simulink model "r4_pfb_fir"  (Simulink 7.0)
settings: Solver=FixedStepDiscrete  SolverMode=SingleTasking  StartTime=0.0  StopTime=10.0  RelTol=1e-3
undefined symbols (not defined in the file): pfb_coefs
libraries: xbsIndex_r4 x385, xps_library x1
(part 2 of 27)

== system r4_pfb_fir/fir_1 ==
  in : Inport  OutDataType=sfix(16)  OutScaling=2^0
  sync_in : Inport  Port=2  OutDataType=sfix(16)  OutScaling=2^0
  Constant : xbsIndex_r4/Constant  arith_type=Unsigned  const=0  n_bits=34  bin_pt=0  explicit_period=on  period=1  equ=P=C  opselect=C  inp2=PCIN>>17  opr=+  inp1=P  carry=CIN  dbl_ovrd=off  block_type=constant
  fir_quantize : Subsystem  mask(FIR Filter Quantizer){n_bits_s=17, bin_pt_s=15, n_bits_o=9, bin_pt_o=7}
      mask prompts: n_bits_s "Number of Bits In"; bin_pt_s "Binary Point In"; n_bits_o "Number of Bits Out"; bin_pt_o "Binary Point Out"
      mask help: A Finite Impluse Response Filter ouput quantizer. This FIR filter output quantizer rounds the sum_in value to the precision specified by n_bits and bin_pt. Overflow wraps, but quantization rounds to even if input binary point is greater than output binary point, otherwise quantization tuncates.
      settings: AttributesFormatString=|
      | 17_15 in
      | 9_7 out
      | round even
      mask Help:
      | <pre>
      | Description::
      | 
      | A Finite Impluse Response Filter ouput quantizer.  This FIR filter output quantizer
      | rounds the sum_in value to the precision specified by n_bits and bin_pt.
      | 
      | Overflow wraps, but quantization rounds to even if input binary point is greater
      | than output binary point, otherwise quantization tuncates.
      | 
      | Mask Parameters::
      | 
      | Number of Bits In (n_bits_s): Specifies the width of the sum_in input.
      | 
      | Binary Point In (bin_pt_s): Specifies the binary point of the sum_in input.
      | 
      | Number of Bits Out (n_bits_o): Specifies the width of the output (overflow wraps).
      | 
      | Binary Point Out (bin_pt_o): Specifies the binary point of the output (quantization rounds to even
      | if input binary point is greater than output binary point, othersie quantization truncates).
      | </pre>
  fir_tap_1 : Subsystem  mask(FIR Filter Tap (Real Coefficients)){delay=1024, coef=[7.55822333239443e-005;0.000226337373781674;0.000376546527419557;0.000526209439676531;0.000675325864794748;0.000823895565799559;0.000971918314479012;0.00111939389136366;0.00126632208570627;0.00141270269546109;0.00155853552726339;0.00170382039640892;0.00184855712683285;0.00199274555108931;0.00213638551033019;0.0022794768542842;0.00242201944123601;0.00256401313800475;0.00270545781992298;0.00284635337081542;0.00298669968297734;0.00312649665715319;0.00326574420251518;0.00340444223664131;0.00354259068549404;0.00368018948339813;0.00381723857301899;0.00395373790534074;0.00408968743964404;0.00422508714348402;0.00435993699266828;0.00449423697123439;0.00462798707142765;0.00476118729367882;0.00489383764658139;0.00502593814686929;0.00515748881939405;0.00528848969710218;0.00541894082101253;0.00554884224019323;0.00567819401173886;0.00580699620074764;0.00593524888029807;0.006062952131426;0.0061901060431015;0.00631671071220536;0.00644276624350604;0.00656827274963604;0.00669323035106852;0.00681763917609391;0.00694149936079604;0.00706481104902866;0.00718757439239176;0.00730978955020755;0.00743145668949677;0.00755257598495482;0.00767314761892755;0.00779317178138749;0.00791264866990946;0.00803157848964654;0.00814996145330591;0.00826779778112436;0.00838508770084402;0.00850183144768805;0.00861802926433593;0.00873368140089908;0.00884878811489629;0.00896334967122888;0.00907736634215623;0.00919083840727075;0.00930376615347321;0.0094161498749479;0.00952798987313748;0.00963928645671813;0.00975003994157455;0.00986025065077467;0.00996991891454458;0.0100790450702434;0.0101876294623378;0.0102956724423769;0.0104031743689668;0.010510135607745;0.0106165565313551;0.0107224375194214;0.0108277789585228;0.010932581242168;0.0110368447707688;0.0111405699516152;0.0112437571988492;0.0113464069334393;0.0114485195831541;0.0115500955825369;0.0116511353728793;0.0117516394021958;0.0118516081251968;0.0119510420032635;0.012049941504421;0.0121483071033125;0.0122461392811728;0.0123434385258024;0.0124402053315406;0.0125364401992397;0.0126321436362382;0.0127273161563346;0.0128219582797607;0.0129160705331552;0.0130096534495371;0.013102707568279;0.0131952334350806;0.0132872316019417;0.013378702627136;0.0134696470751837;0.0135600655168253;0.0136499585289943;0.0137393266947904;0.0138281706034528;0.0139164908503332;0.0140042880368685;0.0140915627705541;0.0141783156649169;0.0142645473394878;0.0143502584197752;0.014435449537237;0.0145201213292544;0.0146042744391039;0.0146879095159304;0.0147710272147199;0.014853628196272;0.014935713127173;0.0150172826797681;0.0150983375321339;0.0151788783680517;0.0152589058769791;0.0153384207540233;0.0154174236999132;0.0154959154209719;0.0155738966290892;0.015651368041694;0.0157283303817268;0.0158047843776117;0.0158807307632293;0.0159561702778886;0.0160311036662993;0.0161055316785444;0.016179455070052;0.0162528746015679;0.0163257910391276;0.0163982051540287;0.0164701177228029;0.0165415295271879;0.0166124413541001;0.0166828539956064;0.016752768248896;0.0168221849162531;0.0168911048050285;0.0169595287276116;0.0170274575014029;0.0170948919487855;0.0171618328970972;0.0172282811786028;0.0172942376304655;0.0173597030947194;0.0174246784182411;0.0174891644527217;0.0175531620546388;0.0176166720852282;0.0176796954104559;0.01774223290099;0.0178042854321725;0.0178658538839913;0.0179269391410516;0.0179875420925484;0.0180476636322377;0.0181073046584087;0.0181664660738554;0.0182251487858485;0.0182833537061072;0.018341081750771;0.0183983338403711;0.018455110899803;0.0185114138582973;0.0185672436493922;0.0186226012109047;0.0186774874849029;0.0187319034176773;0.0187858499597128;0.0188393280656603;0.0188923386943085;0.0189448828085557;0.0189969613753813;0.0190485753658179;0.0190997257549227;0.0191504135217495;0.0192006396493202;0.0192504051245967;0.0192997109384527;0.019348558085645;0.0193969475647859;0.0194448803783146;0.0194923575324687;0.0195393800372564;0.0195859489064282;0.0196320651574482;0.0196777298114666;0.0197229438932907;0.0197677084313573;0.0198120244577041 ...(+15786 chars)], n_bits_c=9, bin_pt_c=8, n_bits_d=8, bin_pt_d=7, n_bits_s=17, bin_pt_s=15, coef_bram=on, delay_bram=on, mult_latency=3, add_latency=1, add_bypass=on}
      mask prompts: delay "Tap Delay"; coef "Tap Coefficient(s)"; n_bits_c "Number of Coefficient Bits"; bin_pt_c "Coefficient Binary Point"; n_bits_d "Number of Data Bits"; bin_pt_d "Data Binary Point"; n_bits_s "Number of Sum Bits"; bin_pt_s "Sum Binary Point"; coef_bram "Use BRAM for Coefficients"; delay_bram "Use BRAM for Delay"; mult_latency "Multiplier Latency"; add_latency "Adder Latency"; add_bypass "Bypass Adder"
      mask help: A Finite Impluse Response Filter tap with real coefficients. This FIR filter tap does not have provisions for folding the input sequence to improve multiplier efficiency, so it is suboptimal for "regular" (i.e. non-WOLA) FIR filters. It is intended primarily for WOLA (Weighted OverLap Add) FIR filters.
      settings: AttributesFormatString=|
      | delay 1024 in bram
      | 1024 coefs in bram\nno adder
      mask Help:
      | <pre>
      | Description::
      | 
      | A Finite Impluse Response Filter tap with real coefficients.
      | 
      | This Finite Impluse Response Filter tap is designed to be daisy chained together
      | to form a multi-tap FIR filter.  This FIR filter tap does not have provisions for folding the input
      | sequence to improve multiplier efficiency, so it is suboptimal for "regular" (i.e. non-WOLA)
      | FIR filters.  It is intended primarily for WOLA (Weighted OverLap Add) FIR filters.
      | 
      | Mask Parameters::
      | 
      | Tap Delay (delay):  The inter-tap delay (the N in "z^-N").  For a regular FIR filter, this will be 1.
      | 
      | Tap Coefficiant(s) (coef): The coefficient(s) for this tap.  For a regular FIR filter, this will be a
      | single number.  For a WOLA (Weighted OverLap Add) filter, this will be a vector of numbers.
      | Usually, delay==length(coef), but this is not required.  These should be specified as doubles.
      | They will be rounded and saturated according to the specified number of bits (n_bits_c) and
      | binary point (bin_pt_c).
      | 
      | Number of Coefficient Bits (n_bits_c): The number of bits used for the fixed point binary
      | representation of the coefficient(s).
      | 
      | Coefficient Binary Point (bin_pt_c): The binary point of the fixed point binary representation
      | of the coefficient(s).
      | 
      | Number of Data Bits (n_bits_d): The number of bits for real/imaginary components of the data.
      | 
      | Data Binary Point (bin_pt_d): The binary point for real/imaginary components of the data.
      | 
      | Number of Sum Bits (n_bits_s): Specifies the width of the sum (overflow wraps).
      | 
      | Sum Binary Point (bin_pt_s): Specifies the binary point of the sum (quantization truncates).
      | 
      | Use BRAM for Delay (delay_bram): Check this checkbox to implement the delay using BRAM.
      | If unchecked, the delay will be implemented using SLR16 elements (i.e. slices).
      | 
      | Use BRAM for Coefficients (coef_bram): Check this checkbox to store the coefficients in BRAM.
      | If unchecked, the coefficients will be stored in distributed memory (i.e. slices).
      | This is only relevant is length(coef) is greater than 1; otherwise, a constant block is used.
      | 
      | Multiplier Latency (mult_latency): Latency to use for the underlying multiplier.
      | 
      | Adder Latency (add_latency): Latency to use for the underlying adder.
      | 
      | Adder Bypass (add_bypass): Check this checkbox to bypass the adder.
      | Typically used for the first tap of a multi-tap FIR filter.
      | </pre>
  fir_tap_2 : Subsystem  mask(FIR Filter Tap (Real Coefficients)){delay=1024, coef=[-0.000375660323525046;-0.00112528207646786;-0.00187263770065757;-0.00261772609063303;-0.00336054616203061;-0.00410109685156988;-0.00483937711704019;-0.00557538593728603;-0.00630912231219222;-0.00704058526266978;-0.00776977383064064;-0.00849668707902262;-0.00922132409171369;-0.00994368397357705;-0.0106637658504249;-0.0113815688690025;-0.0120970921969721;-0.0128103350228962;-0.0135212965562215;-0.0142299760272615;-0.0149363726871797;-0.0156404858079725;-0.0163423146824514;-0.0170418586242254;-0.0177391169676835;-0.0184340890679761;-0.0191267743009973;-0.0198171720633655;-0.0205052817724058;-0.0211911028661302;-0.0218746348032188;-0.0225558770630009;-0.0232348291454347;-0.0239114905710882;-0.0245858608811188;-0.0252579396372536;-0.0259277264217688;-0.0265952208374693;-0.0272604225076676;-0.0279233310761635;-0.0285839462072226;-0.0292422675855545;-0.0298982949162921;-0.0305520279249694;-0.0312034663574997;-0.031852609980153;-0.0324994585795345;-0.0331440119625613;-0.0337862699564402;-0.0344262324086442;-0.0350638991868898;-0.0356992701791137;-0.0363323452934489;-0.0369631244582015;-0.0375916076218262;-0.0382177947529027;-0.0388416858401109;-0.0394632808922069;-0.0400825799379981;-0.0406995830263182;-0.0413142902260021;-0.0419267016258609;-0.0425368173346564;-0.0431446374810749;-0.0437501622137022;-0.0443533917009969;-0.0449543261312647;-0.0455529657126312;-0.0461493106730163;-0.0467433612601067;-0.047335117741329;-0.0479245804038229;-0.0485117495544134;-0.0490966255195838;-0.0496792086454471;-0.0502594992977191;-0.0508374978616896;-0.0514132047421944;-0.0519866203635867;-0.0525577451697087;-0.0531265796238626;-0.0536931242087811;-0.0542573794265993;-0.0548193457988244;-0.0553790238663066;-0.0559364141892089;-0.0564915173469777;-0.0570443339383125;-0.0575948645811356;-0.0581431099125613;-0.058689070588866;-0.0592327472854569;-0.0597741406968409;-0.0603132515365938;-0.0608500805373288;-0.0613846284506648;-0.0619168960471949;-0.0624468841164546;-0.0629745934668896;-0.0635000249258237;-0.064023179339426;-0.0645440575726791;-0.0650626605093458;-0.0655789890519362;-0.0660930441216749;-0.0666048266584676;-0.0671143376208679;-0.067621577986043;-0.0681265487497408;-0.0686292509262558;-0.0691296855483946;-0.0696278536674418;-0.0701237563531258;-0.0706173946935843;-0.071108769795329;-0.071597882783211;-0.0720847348003859;-0.0725693270082785;-0.0730516605865468;-0.0735317367330474;-0.0740095566637989;-0.0744851216129466;-0.0749584328327259;-0.0754294915934268;-0.0758982991833568;-0.0763648569088048;-0.0768291660940042;-0.0772912280810962;-0.0777510442300928;-0.0782086159188393;-0.0786639445429775;-0.0791170315159078;-0.0795678782687517;-0.0800164862503141;-0.0804628569270452;-0.0809069917830028;-0.0813488923198131;-0.0817885600566336;-0.0822259965301136;-0.0826612032943558;-0.0830941819208773;-0.0835249339985711;-0.0839534611336661;-0.0843797649496887;-0.0848038470874227;-0.0852257092048699;-0.0856453529772106;-0.0860627800967632;-0.0864779922729447;-0.0868909912322302;-0.0873017787181127;-0.0877103564910625;-0.0881167263284868;-0.0885208900246886;-0.0889228493908263;-0.0893226062548723;-0.0897201624615717;-0.0901155198724016;-0.0905086803655288;-0.0908996458357691;-0.0912884181945446;-0.0916749993698427;-0.0920593913061736;-0.0924415959645284;-0.0928216153223364;-0.0931994513734234;-0.0935751061279683;-0.0939485816124612;-0.09431987986966;-0.0946890029585477;-0.0950559529542894;-0.0954207319481889;-0.0957833420476455;-0.0961437853761105;-0.0965020640730433;-0.0968581802938682;-0.0972121362099301;-0.0975639340084509;-0.0979135758924848;-0.0982610640808748;-0.0986064008082076;-0.0989495883247697;-0.0992906288965024;-0.0996295248049575;-0.0999662783472516;-0.100300891836022;-0.100633367599381;-0.100963707980872;-0.101291915339421;-0.101617992049296;-0.101941940500055;-0.102263763096507;-0.102583462258662;-0.102901040421687;-0.103216500035856;-0.103529843566511;-0.103841073494009;-0.104150192313679;-0.104457202535775;-0.104762106685429 ...(+16057 chars)], n_bits_c=9, bin_pt_c=8, n_bits_d=8, bin_pt_d=7, n_bits_s=17, bin_pt_s=15, coef_bram=on, delay_bram=on, mult_latency=3, add_latency=1, add_bypass=off}
      mask prompts: delay "Tap Delay"; coef "Tap Coefficient(s)"; n_bits_c "Number of Coefficient Bits"; bin_pt_c "Coefficient Binary Point"; n_bits_d "Number of Data Bits"; bin_pt_d "Data Binary Point"; n_bits_s "Number of Sum Bits"; bin_pt_s "Sum Binary Point"; coef_bram "Use BRAM for Coefficients"; delay_bram "Use BRAM for Delay"; mult_latency "Multiplier Latency"; add_latency "Adder Latency"; add_bypass "Bypass Adder"
      mask help: A Finite Impluse Response Filter tap with real coefficients. This FIR filter tap does not have provisions for folding the input sequence to improve multiplier efficiency, so it is suboptimal for "regular" (i.e. non-WOLA) FIR filters. It is intended primarily for WOLA (Weighted OverLap Add) FIR filters.
      settings: AttributesFormatString=|
      | delay 1024 in bram
      | 1024 coefs in bram
      mask Help:
      | <pre>
      | Description::
      | 
      | A Finite Impluse Response Filter tap with real coefficients.
      | 
      | This Finite Impluse Response Filter tap is designed to be daisy chained together
      | to form a multi-tap FIR filter.  This FIR filter tap does not have provisions for folding the input
      | sequence to improve multiplier efficiency, so it is suboptimal for "regular" (i.e. non-WOLA)
      | FIR filters.  It is intended primarily for WOLA (Weighted OverLap Add) FIR filters.
      | 
      | Mask Parameters::
      | 
      | Tap Delay (delay):  The inter-tap delay (the N in "z^-N").  For a regular FIR filter, this will be 1.
      | 
      | Tap Coefficiant(s) (coef): The coefficient(s) for this tap.  For a regular FIR filter, this will be a
      | single number.  For a WOLA (Weighted OverLap Add) filter, this will be a vector of numbers.
      | Usually, delay==length(coef), but this is not required.  These should be specified as doubles.
      | They will be rounded and saturated according to the specified number of bits (n_bits_c) and
      | binary point (bin_pt_c).
      | 
      | Number of Coefficient Bits (n_bits_c): The number of bits used for the fixed point binary
      | representation of the coefficient(s).
      | 
      | Coefficient Binary Point (bin_pt_c): The binary point of the fixed point binary representation
      | of the coefficient(s).
      | 
      | Number of Data Bits (n_bits_d): The number of bits for real/imaginary components of the data.
      | 
      | Data Binary Point (bin_pt_d): The binary point for real/imaginary components of the data.
      | 
      | Number of Sum Bits (n_bits_s): Specifies the width of the sum (overflow wraps).
      | 
      | Sum Binary Point (bin_pt_s): Specifies the binary point of the sum (quantization truncates).
      | 
      | Use BRAM for Delay (delay_bram): Check this checkbox to implement the delay using BRAM.
      | If unchecked, the delay will be implemented using SLR16 elements (i.e. slices).
      | 
      | Use BRAM for Coefficients (coef_bram): Check this checkbox to store the coefficients in BRAM.
      | If unchecked, the coefficients will be stored in distributed memory (i.e. slices).
      | This is only relevant is length(coef) is greater than 1; otherwise, a constant block is used.
      | 
      | Multiplier Latency (mult_latency): Latency to use for the underlying multiplier.
      | 
      | Adder Latency (add_latency): Latency to use for the underlying adder.
      | 
      | Adder Bypass (add_bypass): Check this checkbox to bypass the adder.
      | Typically used for the first tap of a multi-tap FIR filter.
      | </pre>
  fir_tap_3 : Subsystem  mask(FIR Filter Tap (Real Coefficients)){delay=1024, coef=[0.999999547662946;0.999995928971626;0.999988691616268;0.999977835651433;0.999963361158965;0.999945268247983;0.999923557054889;0.99989822774336;0.999869280504348;0.999836715556079;0.999800533144051;0.99976073354103;0.999717317047049;0.999670283989403;0.999619634722648;0.999565369628596;0.999507489116311;0.999445993622108;0.999380883609544;0.999312159569415;0.999239822019754;0.999163871505822;0.999084308600105;0.999001133902306;0.998914348039344;0.998823951665339;0.998729945461616;0.99863233013669;0.998531106426262;0.998426275093213;0.998317836927595;0.998205792746621;0.998090143394661;0.997970889743233;0.99784803269099;0.997721573163716;0.997591512114315;0.997457850522799;0.997320589396285;0.997179729768976;0.997035272702159;0.99688721928419;0.996735570630482;0.996580327883498;0.996421492212737;0.996259064814724;0.996093046912996;0.99592343975809;0.995750244627533;0.995573462825828;0.99539309568444;0.995209144561783;0.995021610843209;0.994830495940991;0.99463580129431;0.994437528369243;0.994235678658745;0.994030253682635;0.993821254987582;0.993608684147091;0.993392542761483;0.993172832457882;0.992949554890201;0.99272271173912;0.992492304712073;0.992258335543232;0.992020805993488;0.991779717850431;0.991535072928337;0.991286873068149;0.991035120137455;0.990779816030475;0.990520962668036;0.990258561997559;0.989992615993036;0.989723126655011;0.989450096010561;0.989173526113274;0.988893419043231;0.988609776906985;0.988322601837537;0.98803189599432;0.987737661563173;0.987439900756322;0.987138615812356;0.986833808996206;0.986525482599124;0.986213638938657;0.985898280358627;0.985579409229105;0.98525702794639;0.984931138932984;0.984601744637569;0.984268847534979;0.98393245012618;0.983592554938246;0.983249164524326;0.98290228146363;0.982551908361392;0.982198047848854;0.981840702583234;0.9814798752477;0.981115568551347;0.980747785229165;0.980376528042017;0.98000179977661;0.979623603245462;0.979241941286885;0.978856816764947;0.978468232569446;0.978076191615887;0.977680696845445;0.977281751224942;0.976879357746813;0.97647351942908;0.976064239315321;0.975651520474639;0.975235366001631;0.97481577901636;0.974392762664321;0.973966320116415;0.973536454568909;0.973103169243412;0.972666467386842;0.972226352271389;0.971782827194488;0.971335895478783;0.970885560472097;0.970431825547395;0.969974694102756;0.969514169561332;0.969050255371323;0.968582955005935;0.96811227196335;0.967638209766689;0.967160771963981;0.966679962128122;0.966195783856846;0.965708240772684;0.965217336522932;0.964723074779614;0.964225459239442;0.963724493623787;0.963220181678634;0.962712527174551;0.962201533906649;0.961687205694544;0.961169546382321;0.960648559838497;0.960124249955978;0.959596620652025;0.959065675868214;0.958531419570396;0.95799385574866;0.957452988417292;0.956908821614734;0.956361359403548;0.955810605870372;0.955256565125884;0.954699241304754;0.954138638565613;0.953574761091004;0.953007613087343;0.952437198784881;0.951863522437655;0.951286588323455;0.950706400743774;0.950122964023769;0.949536282512219;0.948946360581481;0.948353202627446;0.947756813069498;0.947157196350468;0.946554356936591;0.945948299317464;0.945339028005997;0.944726547538374;0.944110862474005;0.943491977395482;0.942869896908532;0.942244625641977;0.941616168247679;0.940984529400506;0.940349713798277;0.939711726161716;0.939070571234412;0.938426253782768;0.937778778595951;0.937128150485851;0.936474374287031;0.935817454856679;0.935157397074559;0.934494205842967;0.933827886086677;0.933158442752899;0.932485880811225;0.931810205253583;0.931131421094187;0.930449533369489;0.929764547138127;0.929076467480875;0.928385299500598;0.927691048322198;0.92699371909256;0.926293316980511;0.925589847176761;0.924883314893854;0.924173725366119;0.923461083849616;0.922745395622088;0.922026665982904;0.92130490025301;0.920580103774877;0.919852281912448;0.919121440051086;0.918387583597519;0.91765071797979;0.9169108486472;0.916167981070258;0.915422120740627;0.914673273171068;0.913921443895387;0.913166638468382 ...(+14460 chars)], n_bits_c=9, bin_pt_c=8, n_bits_d=8, bin_pt_d=7, n_bits_s=17, bin_pt_s=15, coef_bram=on, delay_bram=on, mult_latency=3, add_latency=1, add_bypass=off}
      mask prompts: delay "Tap Delay"; coef "Tap Coefficient(s)"; n_bits_c "Number of Coefficient Bits"; bin_pt_c "Coefficient Binary Point"; n_bits_d "Number of Data Bits"; bin_pt_d "Data Binary Point"; n_bits_s "Number of Sum Bits"; bin_pt_s "Sum Binary Point"; coef_bram "Use BRAM for Coefficients"; delay_bram "Use BRAM for Delay"; mult_latency "Multiplier Latency"; add_latency "Adder Latency"; add_bypass "Bypass Adder"
      mask help: A Finite Impluse Response Filter tap with real coefficients. This FIR filter tap does not have provisions for folding the input sequence to improve multiplier efficiency, so it is suboptimal for "regular" (i.e. non-WOLA) FIR filters. It is intended primarily for WOLA (Weighted OverLap Add) FIR filters.
      settings: AttributesFormatString=|
      | delay 1024 in bram
      | 1024 coefs in bram
      mask Help:
      | <pre>
      | Description::
      | 
      | A Finite Impluse Response Filter tap with real coefficients.
      | 
      | This Finite Impluse Response Filter tap is designed to be daisy chained together
      | to form a multi-tap FIR filter.  This FIR filter tap does not have provisions for folding the input
      | sequence to improve multiplier efficiency, so it is suboptimal for "regular" (i.e. non-WOLA)
      | FIR filters.  It is intended primarily for WOLA (Weighted OverLap Add) FIR filters.
      | 
      | Mask Parameters::
      | 
      | Tap Delay (delay):  The inter-tap delay (the N in "z^-N").  For a regular FIR filter, this will be 1.
      | 
      | Tap Coefficiant(s) (coef): The coefficient(s) for this tap.  For a regular FIR filter, this will be a
      | single number.  For a WOLA (Weighted OverLap Add) filter, this will be a vector of numbers.
      | Usually, delay==length(coef), but this is not required.  These should be specified as doubles.
      | They will be rounded and saturated according to the specified number of bits (n_bits_c) and
      | binary point (bin_pt_c).
      | 
      | Number of Coefficient Bits (n_bits_c): The number of bits used for the fixed point binary
      | representation of the coefficient(s).
      | 
      | Coefficient Binary Point (bin_pt_c): The binary point of the fixed point binary representation
      | of the coefficient(s).
      | 
      | Number of Data Bits (n_bits_d): The number of bits for real/imaginary components of the data.
      | 
      | Data Binary Point (bin_pt_d): The binary point for real/imaginary components of the data.
      | 
      | Number of Sum Bits (n_bits_s): Specifies the width of the sum (overflow wraps).
      | 
      | Sum Binary Point (bin_pt_s): Specifies the binary point of the sum (quantization truncates).
      | 
      | Use BRAM for Delay (delay_bram): Check this checkbox to implement the delay using BRAM.
      | If unchecked, the delay will be implemented using SLR16 elements (i.e. slices).
      | 
      | Use BRAM for Coefficients (coef_bram): Check this checkbox to store the coefficients in BRAM.
      | If unchecked, the coefficients will be stored in distributed memory (i.e. slices).
      | This is only relevant is length(coef) is greater than 1; otherwise, a constant block is used.
      | 
      | Multiplier Latency (mult_latency): Latency to use for the underlying multiplier.
      | 
      | Adder Latency (add_latency): Latency to use for the underlying adder.
      | 
      | Adder Bypass (add_bypass): Check this checkbox to bypass the adder.
      | Typically used for the first tap of a multi-tap FIR filter.
      | </pre>
  fir_tap_4 : Subsystem  mask(FIR Filter Tap (Real Coefficients)){delay=1024, coef=[0.000376226431598763;0.00113037704120664;0.00188679033646423;0.00264546512738635;0.00340640020282435;0.00416959433045314;0.00493504625675948;0.00570275470702945;0.00647271838533626;0.00724493597452914;0.00801940613622144;0.00879612751077952;0.00957509871731131;0.0103563183536561;0.0111397849963734;0.0119254972007329;0.0127134535007037;0.0135036524089452;0.0142960924167967;0.0150907719942678;0.0158876895900297;0.0166868436314057;0.0174882325243625;0.0182918546535009;0.0190977083820486;0.019905792051851;0.0207161039833637;0.0215286424756441;0.022343405806345;0.0231603922317064;0.0239795999865484;0.0248010272842649;0.0256246723168164;0.026450533254724;0.0272786082470629;0.0281088954214566;0.0289413928840709;0.0297760987196091;0.0306130109913055;0.0314521277409214;0.0322934469887399;0.0331369667335609;0.0339826849526973;0.0348305996019707;0.035680708615707;0.0365330099067331;0.0373875013663734;0.0382441808644464;0.0391030462492619;0.0399640953476175;0.0408273259647971;0.0416927358845677;0.0425603228691775;0.0434300846593541;0.0443020189743029;0.0451761235117054;0.0460523959477181;0.0469308339369715;0.0478114351125697;0.0486941970860893;0.0495791174475793;0.0504661937655611;0.0513554235870291;0.0522468044374499;0.0531403338207642;0.0540360092193872;0.0549338280942094;0.055833787884598;0.0567358860083988;0.0576401198619378;0.0585464868200229;0.0594549842359465;0.0603656094414881;0.0612783597469165;0.062193232440993;0.0631102247909746;0.0640293340426176;0.0649505574201807;0.0658738921264291;0.066799335342639;0.0677268842286013;0.0686565359226264;0.069588287541549;0.0705221361807334;0.0714580789140785;0.0723961127940227;0.0733362348515507;0.0742784420961991;0.0752227315160621;0.0761691000777984;0.0771175447266376;0.0780680623863875;0.0790206499594406;0.0799753043267821;0.0809320223479969;0.081890800861278;0.0828516366834338;0.0838145266098974;0.0847794674147343;0.0857464558506515;0.0867154886490061;0.0876865625198155;0.0886596741517658;0.0896348202122217;0.0906119973472373;0.091591202181565;0.0925724313186671;0.0935556813407251;0.094540948808652;0.0955282302621025;0.0965175222194845;0.0975088211779706;0.0985021236135104;0.0994974259808421;0.100494724713505;0.10149401622385;0.102495296903059;0.103498563121147;0.104503811226986;0.105511037548312;0.106520238391741;0.107531410042783;0.108544548765853;0.109559650804292;0.110576712380376;0.111595729695331;0.112616698929352;0.113639616241614;0.114664477770291;0.11569127963257;0.116720017924666;0.117750688721843;0.118783288078423;0.11981781202781;0.120854256582503;0.121892617734113;0.122932891453382;0.123975073690202;0.125019160373628;0.126065147411903;0.12711303069247;0.128162806081993;0.129214469426379;0.13026801655079;0.131323443259671;0.132380745336762;0.133439918545122;0.134500958627148;0.135563861304595;0.136628622278597;0.137695237229687;0.138763701817818;0.139834011682386;0.140906162442248;0.141980149695748;0.143055969020734;0.144133615974584;0.145213086094228;0.146294374896168;0.147377477876504;0.148462390510953;0.149549108254878;0.150637626543306;0.151727940790955;0.152820046392257;0.153913938721383;0.155009613132265;0.156107064958625;0.157206289513996;0.158307282091748;0.159410037965114;0.160514552387217;0.161620820591094;0.162728837789721;0.163838599176042;0.164950099922995;0.166063335183536;0.167178300090671;0.168294989757478;0.169413399277137;0.170533523722959;0.171655358148411;0.172778897587147;0.173904137053034;0.175031071540182;0.176159696022971;0.177290005456083;0.178421994774532;0.179555658893686;0.180690992709306;0.181827991097572;0.182966648915113;0.184106960999035;0.185248922166959;0.186392527217044;0.187537770928023;0.188684648059233;0.189833153350645;0.190983281522898;0.192135027277332;0.193288385296015;0.194443350241782;0.195599916758264;0.196758079469921;0.197917832982076;0.199079171880949;0.200242090733689;0.201406584088409;0.202572646474221;0.203740272401268;0.204909456360757;0.206080192825002;0.207252476247449;0.208426301062716;0.209601661686629 ...(+14467 chars)], n_bits_c=9, bin_pt_c=8, n_bits_d=8, bin_pt_d=7, n_bits_s=17, bin_pt_s=15, coef_bram=on, delay_bram=on, mult_latency=3, add_latency=1, add_bypass=off}
      mask prompts: delay "Tap Delay"; coef "Tap Coefficient(s)"; n_bits_c "Number of Coefficient Bits"; bin_pt_c "Coefficient Binary Point"; n_bits_d "Number of Data Bits"; bin_pt_d "Data Binary Point"; n_bits_s "Number of Sum Bits"; bin_pt_s "Sum Binary Point"; coef_bram "Use BRAM for Coefficients"; delay_bram "Use BRAM for Delay"; mult_latency "Multiplier Latency"; add_latency "Adder Latency"; add_bypass "Bypass Adder"
      mask help: A Finite Impluse Response Filter tap with real coefficients. This FIR filter tap does not have provisions for folding the input sequence to improve multiplier efficiency, so it is suboptimal for "regular" (i.e. non-WOLA) FIR filters. It is intended primarily for WOLA (Weighted OverLap Add) FIR filters.
      settings: AttributesFormatString=|
      | delay 1024 in bram
      | 1024 coefs in bram
      mask Help:
      | <pre>
      | Description::
      | 
      | A Finite Impluse Response Filter tap with real coefficients.
      | 
      | This Finite Impluse Response Filter tap is designed to be daisy chained together
      | to form a multi-tap FIR filter.  This FIR filter tap does not have provisions for folding the input
      | sequence to improve multiplier efficiency, so it is suboptimal for "regular" (i.e. non-WOLA)
      | FIR filters.  It is intended primarily for WOLA (Weighted OverLap Add) FIR filters.
      | 
      | Mask Parameters::
      | 
      | Tap Delay (delay):  The inter-tap delay (the N in "z^-N").  For a regular FIR filter, this will be 1.
      | 
      | Tap Coefficiant(s) (coef): The coefficient(s) for this tap.  For a regular FIR filter, this will be a
      | single number.  For a WOLA (Weighted OverLap Add) filter, this will be a vector of numbers.
      | Usually, delay==length(coef), but this is not required.  These should be specified as doubles.
      | They will be rounded and saturated according to the specified number of bits (n_bits_c) and
      | binary point (bin_pt_c).
      | 
      | Number of Coefficient Bits (n_bits_c): The number of bits used for the fixed point binary
      | representation of the coefficient(s).
      | 
      | Coefficient Binary Point (bin_pt_c): The binary point of the fixed point binary representation
      | of the coefficient(s).
      | 
      | Number of Data Bits (n_bits_d): The number of bits for real/imaginary components of the data.
      | 
      | Data Binary Point (bin_pt_d): The binary point for real/imaginary components of the data.
      | 
      | Number of Sum Bits (n_bits_s): Specifies the width of the sum (overflow wraps).
      | 
      | Sum Binary Point (bin_pt_s): Specifies the binary point of the sum (quantization truncates).
      | 
      | Use BRAM for Delay (delay_bram): Check this checkbox to implement the delay using BRAM.
      | If unchecked, the delay will be implemented using SLR16 elements (i.e. slices).
      | 
      | Use BRAM for Coefficients (coef_bram): Check this checkbox to store the coefficients in BRAM.
      | If unchecked, the coefficients will be stored in distributed memory (i.e. slices).
      | This is only relevant is length(coef) is greater than 1; otherwise, a constant block is used.
      | 
      | Multiplier Latency (mult_latency): Latency to use for the underlying multiplier.
      | 
      | Adder Latency (add_latency): Latency to use for the underlying adder.
      | 
      | Adder Bypass (add_bypass): Check this checkbox to bypass the adder.
      | Typically used for the first tap of a multi-tap FIR filter.
      | </pre>
  fir_tap_5 : Subsystem  mask(FIR Filter Tap (Real Coefficients)){delay=1024, coef=[-7.57186305694141e-005;-0.000227564945670749;-0.000379956430889435;-0.000532892796251757;-0.000686373742881339;-0.000840398962979647;-0.000994968139806186;-0.00115008094765919;-0.00130573705185642;-0.00146193610871559;-0.00161867776553536;-0.00177596166057639;-0.00193378742304204;-0.0020921546730598;-0.0022510630216622;-0.00241051207076825;-0.00257050141316491;-0.00273103063248833;-0.00289209930320557;-0.00305370699059638;-0.00321585325073467;-0.00337853763047057;-0.00354175966741245;-0.00370551888990871;-0.00386981481703025;-0.00403464695855241;-0.00420001481493748;-0.00436591787731722;-0.0045323556274752;-0.00469932753782952;-0.00486683307141569;-0.00503487168186923;-0.00520344281340873;-0.00537254590081901;-0.00554218036943399;-0.00571234563512023;-0.00588304110426002;-0.00605426617373492;-0.00622602023090949;-0.00639830265361464;-0.00657111281013151;-0.00674445005917552;-0.00691831374988003;-0.00709270322178053;-0.00726761780479901;-0.00744305681922785;-0.00761901957571464;-0.00779550537524631;-0.0079725135091339;-0.00815004325899737;-0.00832809389675017;-0.0085066646845843;-0.00868575487495546;-0.00886536371056795;-0.00904549042435999;-0.00922613423948933;-0.00940729436931827;-0.0095889700173997;-0.00977116037746245;-0.00995386463339719;-0.0101370819592425;-0.0103208115191707;-0.010505052467474;-0.0106898039485508;-0.0108750650968923;-0.0110608350370682;-0.0112471128837145;-0.011433897741519;-0.0116211887052088;-0.0118089848595372;-0.0119972852792704;-0.0121860890291751;-0.0123753951640054;-0.0125652027284904;-0.0127555107573218;-0.0129463182751411;-0.013137624296528;-0.0133294278259877;-0.0135217278579391;-0.013714523376703;-0.0139078133564902;-0.0141015967613896;-0.0142958725453573;-0.0144906396522044;-0.0146858970155864;-0.0148816435589916;-0.01507787819573;-0.0152745998289226;-0.0154718073514906;-0.0156694996461444;-0.0158676755853733;-0.016066334031435;-0.016265473836345;-0.0164650938418669;-0.016665192879502;-0.0168657697704791;-0.0170668233257453;-0.0172683523459559;-0.0174703556214645;-0.0176728319323143;-0.0178757800482282;-0.0180791987285998;-0.0182830867224842;-0.018487442768589;-0.0186922655952659;-0.0188975539205014;-0.0191033064519087;-0.019309521886719;-0.0195161989117731;-0.0197233362035136;-0.0199309324279764;-0.0201389862407831;-0.020347496287133;-0.0205564612017955;-0.0207658796091025;-0.0209757501229411;-0.0211860713467461;-0.0213968418734932;-0.0216080602856917;-0.0218197251553776;-0.022031835044107;-0.0222443885029495;-0.0224573840724814;-0.0226708202827797;-0.0228846956534157;-0.0230990086934489;-0.0233137579014212;-0.0235289417653507;-0.0237445587627263;-0.0239606073605024;-0.0241770860150929;-0.024393993172366;-0.0246113272676396;-0.0248290867256759;-0.025047269960676;-0.0252658753762764;-0.0254849013655432;-0.0257043463109681;-0.0259242085844644;-0.026144486547362;-0.0263651785504042;-0.026586282933743;-0.026807798026936;-0.0270297221489423;-0.0272520536081191;-0.0274747907022183;-0.0276979317183836;-0.0279214749331467;-0.0281454186124251;-0.0283697610115189;-0.0285945003751079;-0.0288196349372498;-0.029045162921377;-0.0292710825402948;-0.0294973919961793;-0.0297240894805752;-0.0299511731743939;-0.0301786412479123;-0.0304064918607708;-0.0306347231619722;-0.03086333328988;-0.0310923203722177;-0.0313216825260677;-0.0315514178578704;-0.0317815244634236;-0.0320120004278819;-0.0322428438257562;-0.0324740527209136;-0.0327056251665774;-0.0329375592053265;-0.0331698528690966;-0.0334025041791795;-0.0336355111462241;-0.0338688717702371;-0.0341025840405833;-0.0343366459359869;-0.0345710554245323;-0.0348058104636656;-0.0350409090001953;-0.0352763489702948;-0.035512128299503;-0.0357482449027266;-0.0359846966842419;-0.036221481537697;-0.036458597346114;-0.0366960419818909;-0.0369338133068049;-0.0371719091720144;-0.0374103274180622;-0.037649065874878;-0.0378881223617824;-0.038127494687489;-0.0383671806501086;-0.0386071780371525;-0.0388474846255361;-0.0390880981815831;-0.039329016461029;-0.0395702372090256 ...(+16053 chars)], n_bits_c=9, bin_pt_c=8, n_bits_d=8, bin_pt_d=7, n_bits_s=17, bin_pt_s=15, coef_bram=on, delay_bram=on, mult_latency=3, add_latency=1, add_bypass=off}
      mask prompts: delay "Tap Delay"; coef "Tap Coefficient(s)"; n_bits_c "Number of Coefficient Bits"; bin_pt_c "Coefficient Binary Point"; n_bits_d "Number of Data Bits"; bin_pt_d "Data Binary Point"; n_bits_s "Number of Sum Bits"; bin_pt_s "Sum Binary Point"; coef_bram "Use BRAM for Coefficients"; delay_bram "Use BRAM for Delay"; mult_latency "Multiplier Latency"; add_latency "Adder Latency"; add_bypass "Bypass Adder"
      mask help: A Finite Impluse Response Filter tap with real coefficients. This FIR filter tap does not have provisions for folding the input sequence to improve multiplier efficiency, so it is suboptimal for "regular" (i.e. non-WOLA) FIR filters. It is intended primarily for WOLA (Weighted OverLap Add) FIR filters.
      settings: AttributesFormatString=|
      | delay 1024 in bram
      | 1024 coefs in bram
      mask Help:
      | <pre>
      | Description::
      | 
      | A Finite Impluse Response Filter tap with real coefficients.
      | 
      | This Finite Impluse Response Filter tap is designed to be daisy chained together
      | to form a multi-tap FIR filter.  This FIR filter tap does not have provisions for folding the input
      | sequence to improve multiplier efficiency, so it is suboptimal for "regular" (i.e. non-WOLA)
      | FIR filters.  It is intended primarily for WOLA (Weighted OverLap Add) FIR filters.
      | 
      | Mask Parameters::
      | 
      | Tap Delay (delay):  The inter-tap delay (the N in "z^-N").  For a regular FIR filter, this will be 1.
      | 
      | Tap Coefficiant(s) (coef): The coefficient(s) for this tap.  For a regular FIR filter, this will be a
      | single number.  For a WOLA (Weighted OverLap Add) filter, this will be a vector of numbers.
      | Usually, delay==length(coef), but this is not required.  These should be specified as doubles.
      | They will be rounded and saturated according to the specified number of bits (n_bits_c) and
      | binary point (bin_pt_c).
      | 
      | Number of Coefficient Bits (n_bits_c): The number of bits used for the fixed point binary
      | representation of the coefficient(s).
      | 
      | Coefficient Binary Point (bin_pt_c): The binary point of the fixed point binary representation
      | of the coefficient(s).
      | 
      | Number of Data Bits (n_bits_d): The number of bits for real/imaginary components of the data.
      | 
      | Data Binary Point (bin_pt_d): The binary point for real/imaginary components of the data.
      | 
      | Number of Sum Bits (n_bits_s): Specifies the width of the sum (overflow wraps).
      | 
      | Sum Binary Point (bin_pt_s): Specifies the binary point of the sum (quantization truncates).
      | 
      | Use BRAM for Delay (delay_bram): Check this checkbox to implement the delay using BRAM.
      | If unchecked, the delay will be implemented using SLR16 elements (i.e. slices).
      | 
      | Use BRAM for Coefficients (coef_bram): Check this checkbox to store the coefficients in BRAM.
      | If unchecked, the coefficients will be stored in distributed memory (i.e. slices).
      | This is only relevant is length(coef) is greater than 1; otherwise, a constant block is used.
      | 
      | Multiplier Latency (mult_latency): Latency to use for the underlying multiplier.
      | 
      | Adder Latency (add_latency): Latency to use for the underlying adder.
      | 
      | Adder Bypass (add_bypass): Check this checkbox to bypass the adder.
      | Typically used for the first tap of a multi-tap FIR filter.
      | </pre>
  fir_tap_6 : Subsystem  mask(FIR Filter Tap (Real Coefficients)){delay=0, coef=[1.30229478472013e-005;3.90815624059165e-005;6.51573367774649e-005;9.12505128142159e-005;0.000117361332654004;0.000143490038707315;0.000169636873644433;0.000195802080382638;0.000221985902073233;0.000248188582088693;0.00027441036400972;0.000300651491612275;0.00032691220885466;0.000353192759864432;0.00037949338892544;0.000405814340464771;0.000432155859039685;0.000458518189324518;0.000484901576097635;0.000511306264228219;0.00053773249866318;0.000564180524413982;0.000590650586543436;0.000617142930152563;0.000643657800367275;0.000670195442325197;0.000696756101162392;0.00072334002200008;0.000749947449931329;0.000776578630007802;0.000803233807226332;0.000829913226515637;0.00085661713272294;0.000883345770600572;0.000910099384792634;0.000936878219821494;0.000963682520074419;0.000990512529790111;0.00101736849304526;0.00104425065374103;0.00107115925558966;0.00109809454210086;0.00112505675656834;0.00115204614205629;0.0011790629413858;0.00120610739712138;0.00123317975155729;0.00126028024670401;0.00128740912427467;0.0013145666256714;0.00134175299197172;0.00136896846391498;0.00139621328188859;0.00142348768591449;0.00145079191563545;0.00147812621030134;0.0015054908087556;0.00153288594942139;0.00156031187028796;0.00158776880889696;0.00161525700232871;0.00164277668718846;0.00167032809959269;0.00169791147515534;0.00172552704897407;0.00175317505561652;0.00178085572910654;0.00180856930291045;0.00183631600992321;0.00186409608245468;0.00189190975221584;0.001919757250305;0.00194763880719397;0.00197555465271432;0.00200350501604353;0.00203149012569121;0.00205951020948525;0.00208756549455806;0.00211565620733274;0.00214378257350922;0.00217194481805049;0.00220014316516874;0.00222837783831153;0.002256649060148;0.00228495705255503;0.00231330203660339;0.00234168423254391;0.00237010385979366;0.00239856113692212;0.00242705628163739;0.00245558951077227;0.0024841610402705;0.00251277108517291;0.00254141985960361;0.00257010757675613;0.00259883444887969;0.00262760068726523;0.00265640650223175;0.00268525210311237;0.00271413769824061;0.00274306349493657;0.00277202969949308;0.00280103651716193;0.00283008415214012;0.00285917280755598;0.00288830268545549;0.00291747398678844;0.00294668691139467;0.00297594165799033;0.00300523842415407;0.00303457740631335;0.00306395879973069;0.00309338279848989;0.00312284959548233;0.00315235938239325;0.00318191234968804;0.00321150868659852;0.00324114858110932;0.00327083221994408;0.00330055978855185;0.00333033147109343;0.00336014745042765;0.00339000790809786;0.00341991302431814;0.0034498629779598;0.00347985794653768;0.00350989810619665;0.00353998363169792;0.0035701146964056;0.00360029147227299;0.00363051412982916;0.00366078283816534;0.00369109776492143;0.00372145907627252;0.00375186693691537;0.00378232151005492;0.00381282295739088;0.00384337143910425;0.00387396711384388;0.00390461013871314;0.00393530066925641;0.00396603885944579;0.00399682486166768;0.00402765882670945;0.0040585409037462;0.00408947124032728;0.00412044998236316;0.00415147727411206;0.00418255325816677;0.00421367807544131;0.00424485186515788;0.00427607476483351;0.00430734691026696;0.00433866843552555;0.00437003947293203;0.00440146015305152;0.00443293060467832;0.00446445095482291;0.00449602132869889;0.00452764184970998;0.00455931263943696;0.00459103381762476;0.00462280550216948;0.00465462780910543;0.00468650085259228;0.0047184247449021;0.00475039959640664;0.00478242551556433;0.00481450260890759;0.00484663098103001;0.00487881073457359;0.00491104197021601;0.00494332478665798;0.00497565928061048;0.00500804554678217;0.00504048367786674;0.00507297376453033;0.00510551589539899;0.0051381101570461;0.00517075663397987;0.00520345540863088;0.00523620656133964;0.0052690101703441;0.00530186631176739;0.00533477505960533;0.00536773648571416;0.00540075065979826;0.00543381764939783;0.00546693751987671;0.00550011033441016;0.00553333615397264;0.00556661503732576;0.00559994704100609;0.00563333221931314;0.00566677062429732;0.0057002623057479;0.00573380731118106;0.00576740568582796 ...(+15802 chars)], n_bits_c=9, bin_pt_c=8, n_bits_d=8, bin_pt_d=7, n_bits_s=17, bin_pt_s=15, coef_bram=on, delay_bram=off, mult_latency=3, add_latency=1, add_bypass=off}
      mask prompts: delay "Tap Delay"; coef "Tap Coefficient(s)"; n_bits_c "Number of Coefficient Bits"; bin_pt_c "Coefficient Binary Point"; n_bits_d "Number of Data Bits"; bin_pt_d "Data Binary Point"; n_bits_s "Number of Sum Bits"; bin_pt_s "Sum Binary Point"; coef_bram "Use BRAM for Coefficients"; delay_bram "Use BRAM for Delay"; mult_latency "Multiplier Latency"; add_latency "Adder Latency"; add_bypass "Bypass Adder"
      mask help: A Finite Impluse Response Filter tap with real coefficients. This FIR filter tap does not have provisions for folding the input sequence to improve multiplier efficiency, so it is suboptimal for "regular" (i.e. non-WOLA) FIR filters. It is intended primarily for WOLA (Weighted OverLap Add) FIR filters.
      settings: AttributesFormatString=|
      | delay 0 in slr
      | 1024 coefs in bram
      mask Help:
      | <pre>
      | Description::
      | 
      | A Finite Impluse Response Filter tap with real coefficients.
      | 
      | This Finite Impluse Response Filter tap is designed to be daisy chained together
      | to form a multi-tap FIR filter.  This FIR filter tap does not have provisions for folding the input
      | sequence to improve multiplier efficiency, so it is suboptimal for "regular" (i.e. non-WOLA)
      | FIR filters.  It is intended primarily for WOLA (Weighted OverLap Add) FIR filters.
      | 
      | Mask Parameters::
      | 
      | Tap Delay (delay):  The inter-tap delay (the N in "z^-N").  For a regular FIR filter, this will be 1.
      | 
      | Tap Coefficiant(s) (coef): The coefficient(s) for this tap.  For a regular FIR filter, this will be a
      | single number.  For a WOLA (Weighted OverLap Add) filter, this will be a vector of numbers.
      | Usually, delay==length(coef), but this is not required.  These should be specified as doubles.
      | They will be rounded and saturated according to the specified number of bits (n_bits_c) and
      | binary point (bin_pt_c).
      | 
      | Number of Coefficient Bits (n_bits_c): The number of bits used for the fixed point binary
      | representation of the coefficient(s).
      | 
      | Coefficient Binary Point (bin_pt_c): The binary point of the fixed point binary representation
      | of the coefficient(s).
      | 
      | Number of Data Bits (n_bits_d): The number of bits for real/imaginary components of the data.
      | 
      | Data Binary Point (bin_pt_d): The binary point for real/imaginary components of the data.
      | 
      | Number of Sum Bits (n_bits_s): Specifies the width of the sum (overflow wraps).
      | 
      | Sum Binary Point (bin_pt_s): Specifies the binary point of the sum (quantization truncates).
      | 
      | Use BRAM for Delay (delay_bram): Check this checkbox to implement the delay using BRAM.
      | If unchecked, the delay will be implemented using SLR16 elements (i.e. slices).
      | 
      | Use BRAM for Coefficients (coef_bram): Check this checkbox to store the coefficients in BRAM.
      | If unchecked, the coefficients will be stored in distributed memory (i.e. slices).
      | This is only relevant is length(coef) is greater than 1; otherwise, a constant block is used.
      | 
      | Multiplier Latency (mult_latency): Latency to use for the underlying multiplier.
      | 
      | Adder Latency (add_latency): Latency to use for the underlying adder.
      | 
      | Adder Bypass (add_bypass): Check this checkbox to bypass the adder.
      | Typically used for the first tap of a multi-tap FIR filter.
      | </pre>
  out : Outport  OutDataType=sfix(16)  OutScaling=2^0
  sync_out : Outport  Port=2  OutDataType=sfix(16)  OutScaling=2^0
  wires:
  in/1 -> fir_tap_1/1(data_in)
  sync_in/1 -> fir_tap_1/3(sync_in)
  fir_tap_1/1(data_out) -> fir_tap_2/1(data_in)
  fir_tap_1/2(sum_out) -> fir_tap_2/2(sum_in)
  fir_tap_1/3(sync_out) -> fir_tap_2/3(sync_in)
  fir_tap_2/1(data_out) -> fir_tap_3/1(data_in)
  fir_tap_2/2(sum_out) -> fir_tap_3/2(sum_in)
  fir_tap_2/3(sync_out) -> fir_tap_3/3(sync_in)
  fir_tap_3/1(data_out) -> fir_tap_4/1(data_in)
  fir_tap_3/2(sum_out) -> fir_tap_4/2(sum_in)
  fir_tap_3/3(sync_out) -> fir_tap_4/3(sync_in)
  fir_tap_4/1(data_out) -> fir_tap_5/1(data_in)
  fir_tap_4/2(sum_out) -> fir_tap_5/2(sum_in)
  fir_tap_4/3(sync_out) -> fir_tap_5/3(sync_in)
  fir_tap_5/1(data_out) -> fir_tap_6/1(data_in)
  fir_tap_5/2(sum_out) -> fir_tap_6/2(sum_in)
  fir_tap_5/3(sync_out) -> fir_tap_6/3(sync_in)
  fir_tap_6/1(data_out) -> fir_quantize/1(data_term)
  fir_tap_6/2(sum_out) -> fir_quantize/2(sum_in)
  fir_tap_6/3(sync_out) -> fir_quantize/3(sync_in)
  fir_quantize/1(sum_out) -> out/1
  fir_quantize/2(sync_out) -> sync_out/1
  Constant/1 -> fir_tap_1/2(sum_in)
